simulink model "R7014E_DoubleTankSim2018b_works_on_A"  (R2018a)
settings: Solver=ode5  StartTime=0.0  StopTime=500  FixedStep=0.02  RelTol=1e-3  EnableMultiTasking=on
undefined symbols (not defined in the file): A, B, C, EqPoint, K
Description:
  | Double tank process simulation model
  | V1.0
  | 
  | Author: Wolfgang Birk, LTU
settings Model: MinMaxOverflowLogging=ForceOff  Creator=wolfgang  LastModifiedBy=anttib-5
settings DataIOCC: LimitDataPoints=on  SaveFormat=Array  SignalLoggingSaveFormat=ModelDataLogs
settings OptimizationCC: ExpressionDepthLimit=2147483647  LifeSpan=inf
settings DebuggingCC: UnderspecifiedInitializationDetection=Classic  MergeDetectMultiDrivingBlocksExec=none  SolverPrmCheckMsg=warning  FcnCallInpInsideContextMsg=warning  StateNameClashWarn=warning  SFUnexpectedBacktrackingDiag=warning  SFNoUnconditionalDefaultTransitionDiag=warning  SFExecutionAtInitializationDiag=none
settings HardwareCC: ProdBitPerPointer=32  ProdBitPerSizeT=32  ProdBitPerPtrDiffT=32  ProdLargestAtomicFloat=None  ProdIntDivRoundTo=Undefined  ProdEndianess=Unspecified  ProdWordSize=32  ProdHWDeviceType=32-bit Generic
settings ModelReferenceCC: PropagateSignalLabelsOutOfModel=off
settings CodeAppCC: StateflowObjectComments=on
settings GRTTargetCC: TargetLangStandard=C89/C90 (ANSI)  GeneratePreprocessorConditionals=Disable all
settings ConfigComp: CovMetricSettings=dw  CovHtmlReporting=on  CovSaveCumulativeToWorkspaceVar=on  CovSaveSingleToWorkspaceVar=on  CovExternalEMLEnable=off

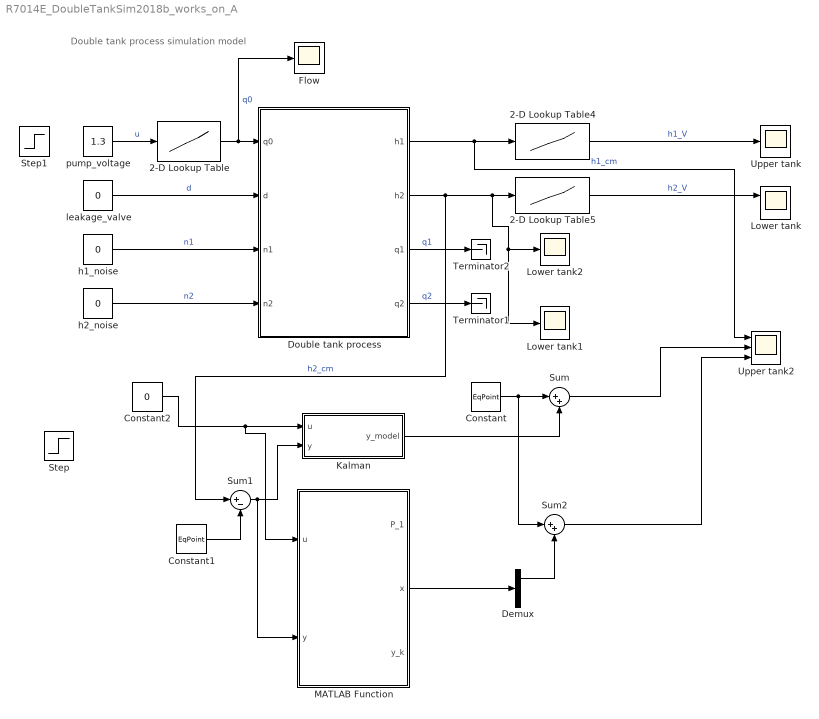
== system R7014E_DoubleTankSim2018b_works_on_A ==
  note: Double tank process simulation model
  2-D Lookup Table : Lookup_n-D  NumberOfTableDimensions=1  BreakpointsForDimension1=x  BreakpointsForDimension2=[1:3]  Table=y  RndMeth=Simplest  InputSameDT=on  mask{x=[0,1,2,3,4,5,6,7,8,9,10], y=[0, 18.86, 28.53, 34.42, 38.82, 42.86, 45.47,47.87, 51, 52, 53.95]}
      mask prompts: x "Values on x-axis"; y "Values on y-axis"
  2-D Lookup Table4 : Lookup_n-D  NumberOfTableDimensions=1  BreakpointsForDimension1=x  BreakpointsForDimension2=[1:3]  Table=y  RndMeth=Simplest  InputSameDT=on  mask{x=[0, 3.4, 5, 6.8, 8.4, 9.7, 11, 12, 13, 14.2, 15.1], y=[0, 0.90, 2.17, 3.54, 4.79, 5.9, 6.997, 7.78, 8.53, 9.395, 9.995]}
      mask prompts: x "Values on x-axis"; y "Values on y-axis"
  2-D Lookup Table5 : Lookup_n-D  NumberOfTableDimensions=1  BreakpointsForDimension1=x  BreakpointsForDimension2=[1:3]  Table=y  RndMeth=Simplest  InputSameDT=on  mask{x=[0, 4.4, 5, 6.1, 7.3, 8.5, 9.6, 10.6, 12, 13.2, 14.7], y=[0, 1.04, 1.71, 2.32, 3.19, 4.11, 5.03, 5.77, 6.68, 7.64, 8.69]}
      mask prompts: x "Values on x-axis"; y "Values on y-axis"
  Constant : Constant  Value=EqPoint
  Constant1 : Constant  Value=EqPoint
  Constant2 : Constant  Value=0
  Demux : Demux  Outputs=2
  Double tank process : Subsystem  mask{At=33, Ao=0.17, hmax=15.5}
      mask prompts: At "Tank area (cm^2)"; Ao "Opening area (cm^2)"; hmax "Tank height (cm)"
      mask help: Double tank process parameters
  Flow : Scope
  Kalman : Subsystem
  Lower tank : Scope  NumInputPorts=2
  Lower tank1 : Scope  NumInputPorts=3
  "Lower tank2 " : Scope
  MATLAB Function : MATLAB Function  TreatAsAtomicUnit=on
  Step : Step  Time=250  After=0.1  SampleTime=0
  Step1 : Step  Time=250  Before=2  After=2.1  SampleTime=0
  Sum : Sum  Inputs=|++
  Sum1 : Sum  Inputs=|+-
  Sum2 : Sum  Inputs=|++
  Terminator1 : Terminator
  Terminator2 : Terminator
  Upper tank : Scope
  Upper tank2 : Scope  NumInputPorts=3
  h1_noise : Constant  Value=0
  h2_noise : Constant  Value=0
  leakage_valve : Constant  Value=0
  pump_voltage : Constant  Value=1.3
  wires:
  2-D Lookup Table4/1 -> Upper tank/1  "h1_V"
  leakage_valve/1 -> Double tank process/2(d)  "d"
  2-D Lookup Table/1 -> Flow/1, Double tank process/1(q0)  "q0"
  Double tank process/1(h1) -> Upper tank2/1, 2-D Lookup Table4/1  "h1_cm"
  Double tank process/2(h2) -> Sum1/1, Lower tank1/2, "Lower tank2 "/1, 2-D Lookup Table5/1  "h2_cm"
  Double tank process/4(q2) -> Terminator1/1  "q2"
  2-D Lookup Table5/1 -> Lower tank/1  "h2_V"
  Double tank process/3(q1) -> Terminator2/1  "q1"
  h1_noise/1 -> Double tank process/3(n1)  "n1"
  h2_noise/1 -> Double tank process/4(n2)  "n2"
  Kalman/1("y_model ") -> Sum/2
  Constant/1 -> Sum2/1, Sum/1
  Constant1/1 -> Sum1/2
  Sum1/1 -> MATLAB Function/2(y), Kalman/2(y)
  Constant2/1 -> MATLAB Function/1(u), Kalman/1(u)
  pump_voltage/1 -> 2-D Lookup Table/1  "u"
  MATLAB Function/2(x) -> Demux/1
  Sum/1 -> Upper tank2/2
  Sum2/1 -> Upper tank2/3
  Demux/1 -> Sum2/2

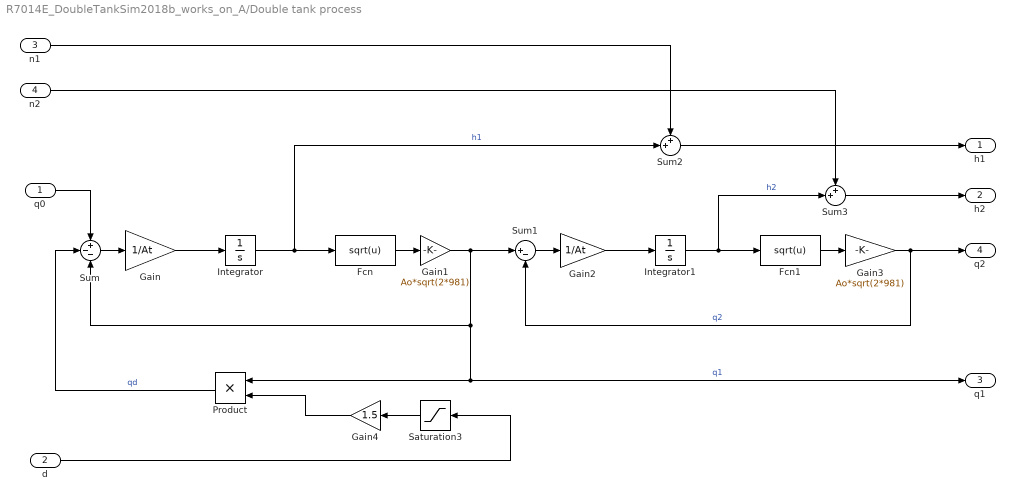
== system R7014E_DoubleTankSim2018b_works_on_A/Double tank process ==
  q0 : Inport
  d : Inport  Port=2
  n1 : Inport  Port=3
  n2 : Inport  Port=4
  Fcn : Fcn  Expr=sqrt(u)
  Fcn1 : Fcn  Expr=sqrt(u)
  Gain : Gain  Gain=1/At
  Gain1 : Gain  Gain=Ao*sqrt(2*981)
  Gain2 : Gain  Gain=1/At
  Gain3 : Gain  Gain=Ao*sqrt(2*981)
  Gain4 : Gain  Gain=1.5
  Integrator : Integrator  InitialCondition=EqPoint  LimitOutput=on  UpperSaturationLimit=hmax  LowerSaturationLimit=0
  Integrator1 : Integrator  InitialCondition=EqPoint  LimitOutput=on  UpperSaturationLimit=hmax  LowerSaturationLimit=0
  Product : Product  RndMeth=Zero
  Saturation3 : Saturate  UpperLimit=1  LowerLimit=0
  Sum : Sum  Inputs=+--
  Sum1 : Sum  Inputs=|+-
  Sum2 : Sum  Inputs=++|
  Sum3 : Sum  Inputs=++|
  h1 : Outport
  h2 : Outport  Port=2
  q1 : Outport  Port=3
  q2 : Outport  Port=4
  wires:
  Sum/1 -> Gain/1
  Gain/1 -> Integrator/1
  Fcn/1 -> Gain1/1
  Gain1/1 -> Sum1/1, Product/1, q1/1, Sum/3  "q1"
  Sum1/1 -> Gain2/1
  Gain2/1 -> Integrator1/1
  Fcn1/1 -> Gain3/1
  Gain3/1 -> Sum1/2, q2/1  "q2"
  q0/1 -> Sum/1
  Integrator/1 -> Sum2/2, Fcn/1  "h1"
  Product/1 -> Sum/2  "qd"
  d/1 -> Saturation3/1
  Integrator1/1 -> Sum3/2, Fcn1/1  "h2"
  Saturation3/1 -> Gain4/1
  Gain4/1 -> Product/2
  Sum2/1 -> h1/1
  n1/1 -> Sum2/1
  Sum3/1 -> h2/1
  n2/1 -> Sum3/1

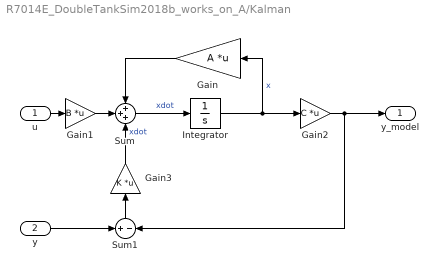
== system R7014E_DoubleTankSim2018b_works_on_A/Kalman ==
  u : Inport
  y : Inport  Port=2
  Gain : Gain  Gain=A  Multiplication=Matrix(K*u)
  Gain1 : Gain  Gain=B  Multiplication=Matrix(K*u)
  Gain2 : Gain  Gain=C  Multiplication=Matrix(K*u)
  Gain3 : Gain  Gain=K  Multiplication=Matrix(K*u)
  Integrator : Integrator
  Sum : Sum  Inputs=+++
  Sum1 : Sum  Inputs=+|-
  "y_model " : Outport
  wires:
  Sum/1 -> Integrator/1  "xdot"
  Integrator/1 -> Gain2/1, Gain/1  "x"
  Gain1/1 -> Sum/2
  u/1 -> Gain1/1
  Gain2/1 -> "y_model "/1, Sum1/2
  y/1 -> Sum1/1
  Sum1/1 -> Gain3/1
  Gain/1 -> Sum/1
  Gain3/1 -> Sum/3  "xdot"

== matlab function R7014E_DoubleTankSim2018b_works_on_A/MATLAB Function ==
  settings: updateMethod=DISCRETE
  data: u input; y input; P_1 output; x output; y_k output
function [P_1,x, y_k] = fcn(u,y)
persistent P_0;
 if isempty(P_0)
        P_0  = [8 8;8 8];
 end
 persistent A_k;
 if isempty(A_k)
        A_k  = [0.991845657443151 0;0.008121005167024 0.991845657417614];
 end
  persistent B_k;
 if isempty(B_k)
        B_k  = [0.001912051102508;7.817036422671138e-06];
 end
  persistent C_k;
 if isempty(C_k)
        C_k  = [0 1];
 end
 persistent N_k;
 if isempty(N_k)
        N_k  = [0 1];
 end
 persistent Q_k;
 if isempty(Q_k)
        Q_k  = [1 0;0 1];
 end
 persistent R_k;
 if isempty(R_k)
        R_k  = 1;
 end
persistent x_0;
 if isempty(x_0)
     x_0 = [0 ; 0];
 end
persistent k_0;
 if isempty(k_0)
    k_0 = 0;
 end
 
x_hat = A_k*x_0+B_k*u;
P = A_k*P_0*A_k'+N_k*Q_k*N_k';

K = P*C_k'*inv(C_k*P*C_k'+R_k);
y_k = y-C_k*x_hat;
x = x_hat+K*y_k;

P_1 = P-K*C_k*P;
